simulink model "ex7_S"  (R2018b)
settings: Solver=VariableStepAuto  StartTime=0.0  StopTime=60  RelTol=1e-3
values from neighbouring files (symbols this model uses):
  A = [-11 -2.5 0;4 0 0;0 0.25 0]    [ex1.m]    (also in ex2.m; ex3.m = sys_s.a; ex4.m = sys_s.A; ex5.m = sys_c.A)
  B = [4 0 0]'    [ex1.m]    (also in ex2.m; ex3.m = sys_s.b; ex4.m = sys_s.B; ex5.m = sys_c.B)
  C = [0 0 5]    [ex1.m]    (also in ex2.m; ex3.m = sys_s.c; ex4.m = sys_s.C; ex5.m = sys_c.C)
  H = -acker(A',C',[lam_o lam_o lam_o*10])'    [ex7.m]    (also in ex8.m; motore.m = -acker(A',C',[lam_o lam_o])'; motore_posizione.m = -acker(A',C',[lam_o1 lam_o2 lam_o1])')
  K = -acker(A,B,lam_d)    [ex1.m]    (also in ex2.m; ex3.m = -acker(A,B,lam_ds); ex4.m; ex5.m)
  k_w = k_d/k_F    [ex2.m]    (also in ex3.m; ex4.m; ex5.m; ex6.m)
settings Model: Creator=michelemaresca  LastModifiedBy=michelemaresca

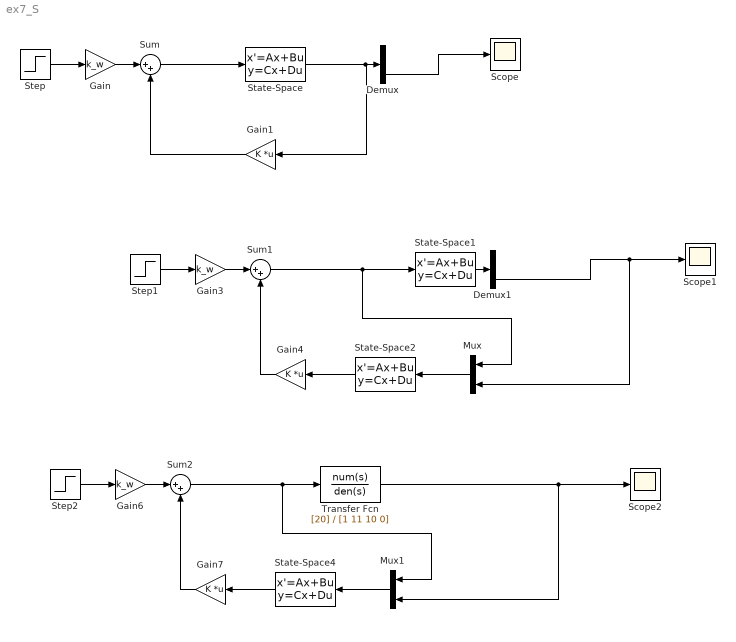
== system ex7_S ==
  Demux : Demux  Outputs=3
  Demux1 : Demux  Outputs=3
  Gain : Gain  Gain=k_w
  Gain1 : Gain  Gain=K  Multiplication=Matrix(K*u)
  Gain3 : Gain  Gain=k_w
  Gain4 : Gain  Gain=K  Multiplication=Matrix(K*u)
  Gain6 : Gain  Gain=k_w
  Gain7 : Gain  Gain=K  Multiplication=Matrix(K*u)
  Mux : Mux  Inputs=2
  Mux1 : Mux  Inputs=2
  Scope : Scope
  Scope1 : Scope
  Scope2 : Scope
  State-Space : StateSpace  A=A  B=B  C=eye(3)  D=zeros(3,1)  InitialCondition=0
  State-Space1 : StateSpace  A=A  B=B  C=eye(3)  D=zeros(3,1)  InitialCondition=0
  State-Space2 : StateSpace  A=A+H*C  B=[B -H]  C=eye(3)  D=zeros(3,2)  InitialCondition=0
  State-Space4 : StateSpace  A=A+H*C  B=[B -H]  C=eye(3)  D=zeros(3,2)  InitialCondition=0
  Step : Step  Time=0  SampleTime=0
  Step1 : Step  Time=0  SampleTime=0
  Step2 : Step  Time=0  SampleTime=0
  Sum : Sum  Inputs=|++
  Sum1 : Sum  Inputs=|++
  Sum2 : Sum  Inputs=|++
  Transfer Fcn : TransferFcn  Numerator=[20]  Denominator=[1 11 10 0]
  wires:
  Step/1 -> Gain/1
  Gain/1 -> Sum/1
  Gain1/1 -> Sum/2
  State-Space/1 -> Demux/1, Gain1/1
  Sum/1 -> State-Space/1
  Gain4/1 -> Sum1/2
  Gain3/1 -> Sum1/1
  State-Space1/1 -> Demux1/1
  Sum1/1 -> Mux/1, State-Space1/1
  Step1/1 -> Gain3/1
  State-Space2/1 -> Gain4/1
  Gain7/1 -> Sum2/2
  Mux1/1 -> State-Space4/1
  State-Space4/1 -> Gain7/1
  Gain6/1 -> Sum2/1
  Step2/1 -> Gain6/1
  Transfer Fcn/1 -> Mux1/2, Scope2/1
  Demux/3 -> Scope/1
  Demux1/3 -> Mux/2, Scope1/1
  Mux/1 -> State-Space2/1
  Sum2/1 -> Transfer Fcn/1, Mux1/1
